simulink model "compressor"  (Simulink 7.4)
settings: Solver=ode45  StartTime=0.0  StopTime=85  RelTol=1e-3
values from neighbouring files (symbols this model uses):
  P_D = 0.9925    [MpcSetup.m]    (also in closedloop_setup.m = 1.12; test_linearization.m = P_D_init + delta_x(end,i))
  Ts = 0.05    [const_sim.m]    (also in test_linearization.m)
  u_out = uoff1(3)    [MpcSetup.m]    (also in closedloop_setup.m)
  x_init_lin = [0.916; 1.145; 0.152; 440; 0]    [closedloop_setup.m]    (also in test_linearization.m = [0.912; 1.17; 0.14; 465; 0])
libraries: dspsrcs4 x3
settings Model: Creator=chkajon  LastModifiedBy=chkajon

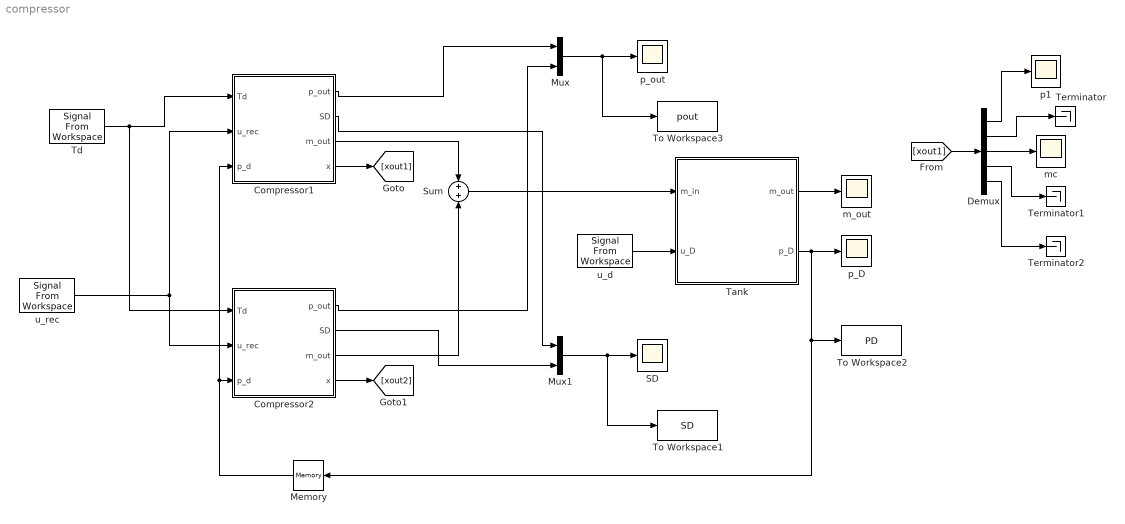
== system compressor ==
  Compressor1 : Subsystem  mask(Compressor){Td_off=0.304, u_in=0.405, u_out=u_out, u_rec=0, t_delay=1}
      mask prompts: Td_off "Torque offset"; u_in "Input valve setting"; u_out "Output valve setting"; u_rec "Recycle valve offset"; t_delay "Time delay"
      mask help: Compressor with tunable inputs.
  Compressor2 : Subsystem  mask(Compressor){Td_off=0.304, u_in=0.405, u_out=u_out, u_rec=0, t_delay=1}
      mask prompts: Td_off "Torque offset"; u_in "Input valve setting"; u_out "Output valve setting"; u_rec "Recycle valve offset"; t_delay "Time delay"
      mask help: Compressor with tunable inputs.
  Demux : Demux  Outputs=5
  Memory : Memory  X0=P_D  LinearizeMemory=on
  Mux : Mux  Inputs=2
  Mux1 : Mux  Inputs=2
  SD : Scope
      settings: YMin=-2.5  YMax=0
  Sum : Sum  OutDataType=fixdt(1, 16)  OutScaling=2^0
  Tank : Subsystem
  Td : dspsrcs4/Signal From Workspace  SystemSampleTime=-1  X=Td  Ts=Ts  nsamps=1  OutputAfterFinalValue=Holding final value  ignoreOrWarnInputAndFrameLengths=off
  Terminator : Terminator
  Terminator1 : Terminator
  Terminator2 : Terminator
  To Workspace1 : ToWorkspace  VariableName=SD  SampleTime=-1  SaveFormat=Structure With Time
  To Workspace2 : ToWorkspace  VariableName=PD  SampleTime=-1  SaveFormat=Structure With Time
  To Workspace3 : ToWorkspace  VariableName=pout  SampleTime=-1  SaveFormat=Structure With Time
  m_out : Scope
      settings: SaveName=ScopeData2
  mc : Scope
      settings: SaveName=ScopeData5
  p1 : Scope
      settings: SaveName=ScopeData4
  p_D : Scope
      settings: YMin=1.01  YMax=1.075  SaveName=ScopeData3
  p_out : Scope
  u_d : dspsrcs4/Signal From Workspace  SystemSampleTime=-1  X=u_d  Ts=Ts  nsamps=1  OutputAfterFinalValue=Holding final value  ignoreOrWarnInputAndFrameLengths=off
  u_rec : dspsrcs4/Signal From Workspace  SystemSampleTime=-1  X=u_rec  Ts=Ts  nsamps=1  OutputAfterFinalValue=Holding final value  ignoreOrWarnInputAndFrameLengths=off
  wires:
  Tank/1(m_out) -> m_out/1
  Tank/2(p_D) -> p_D/1, To Workspace2/1, Memory/1
  Compressor1/1(p_out) -> Mux/1
  Compressor1/2(SD) -> Mux1/1
  Compressor2/1(p_out) -> Mux/2
  Td/1 -> Compressor1/1(Td), Compressor2/1(Td)
  u_rec/1 -> Compressor1/2(u_rec), Compressor2/2(u_rec)
  u_d/1 -> Tank/2(u_D)
  Sum/1 -> Tank/1(m_in)
  Mux1/1 -> SD/1, To Workspace1/1
  Mux/1 -> p_out/1, To Workspace3/1
  Memory/1 -> Compressor1/3(p_d), Compressor2/3(p_d)
  Compressor1/3(m_out) -> Sum/1
  Compressor2/2(SD) -> Mux1/2
  Compressor2/3(m_out) -> Sum/2
  [xout1] -> Demux/1
  Compressor1/4(x) -> [xout1]
  Compressor2/4(x) -> [xout2]
  Demux/1 -> p1/1
  Demux/3 -> mc/1
  Demux/2 -> Terminator/1
  Demux/4 -> Terminator1/1
  Demux/5 -> Terminator2/1

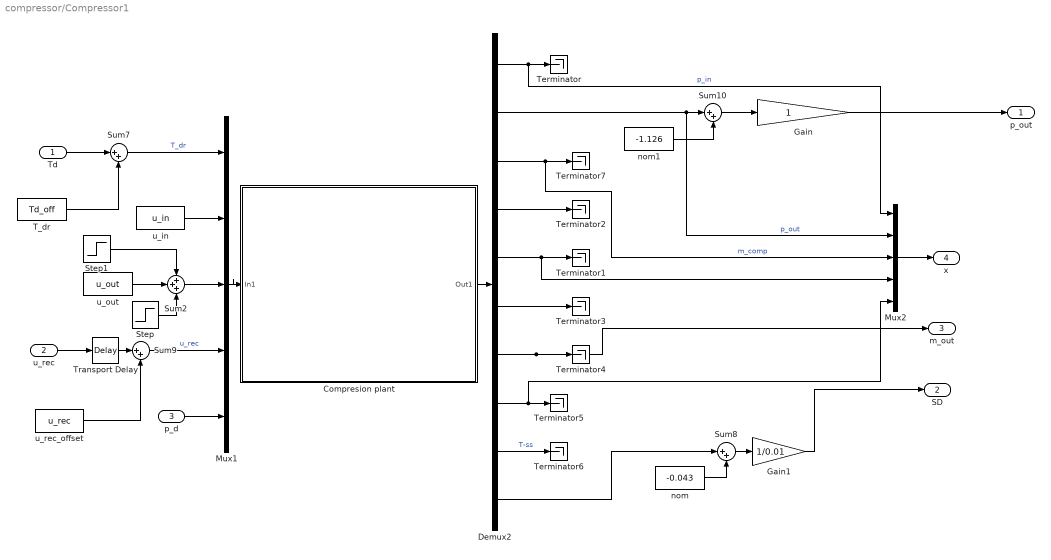
== system compressor/Compressor1 ==
  Td : Inport  OutDataType=fixdt(1, 16)  OutScaling=2^0
  u_rec : Inport  Port=2  OutDataType=fixdt(1, 16)  OutScaling=2^0
  p_d : Inport  Port=3  OutDataType=fixdt(1, 16)  OutScaling=2^0
  Compresion plant : Subsystem
      mask Display: image(imread('comp_plant.jpg'))
  Demux2 : Demux  Outputs=10
  Gain : Gain
  Gain1 : Gain  Gain=1/0.01
  Mux1 : Mux  Inputs=5
  Mux2 : Mux  Inputs=5
  Step : Step  Time=50  After=0  SampleTime=0
  Step1 : Step  Time=100  After=0  SampleTime=0
  Sum{7..10} (4 alike) : Sum  Inputs=|++
  Sum2 : Sum  Inputs=+++
  T_dr : Constant  Value=Td_off
  Terminator{,1..7} (8 alike) : Terminator
  Transport Delay : TransportDelay  DelayTime=t_delay
  nom : Constant  Value=-0.043
  nom1 : Constant  Value=-1.126
  u_in : Constant  Value=u_in
  u_out : Constant  Value=u_out
  u_rec_offset : Constant  Value=u_rec
  p_out : Outport  OutDataType=fixdt(1, 16)  OutScaling=2^0
  SD : Outport  Port=2  OutDataType=fixdt(1, 16)  OutScaling=2^0
  m_out : Outport  Port=3  OutDataType=fixdt(1, 16)  OutScaling=2^0
  x : Outport  Port=4  OutDataType=fixdt(1, 16)  OutScaling=2^0
  wires:
  Mux2/1 -> x/1
  Demux2/9 -> Terminator6/1  "T-ss"
  Sum2/1 -> Mux1/3
  Step/1 -> Sum2/3
  Transport Delay/1 -> Sum9/1
  p_d/1 -> Mux1/5
  Demux2/10 -> Sum8/1
  Gain1/1 -> SD/1
  Td/1 -> Sum7/1
  u_rec_offset/1 -> Sum9/2
  T_dr/1 -> Sum7/2
  Gain/1 -> p_out/1
  nom1/1 -> Sum10/2
  Sum10/1 -> Gain/1
  Demux2/5 -> Mux2/4, Terminator1/1
  Demux2/1 -> Mux2/1, Terminator/1  "p_in"
  Demux2/2 -> Mux2/2, Sum10/1  "p_out"
  Sum8/1 -> Gain1/1
  nom/1 -> Sum8/2
  Sum9/1 -> Mux1/4  "u_rec"
  Sum7/1 -> Mux1/1  "T_dr"
  u_rec/1 -> Transport Delay/1
  u_out/1 -> Sum2/2
  Demux2/7 -> Terminator4/1, m_out/1
  Demux2/8 -> Mux2/5, Terminator5/1
  Demux2/6 -> Terminator3/1
  u_in/1 -> Mux1/2
  Mux1/1 -> Compresion plant/1(In1)
  Compresion plant/1(Out1) -> Demux2/1
  Step1/1 -> Sum2/1
  Demux2/3 -> Mux2/3, Terminator7/1  "m_comp"
  Demux2/4 -> Terminator2/1

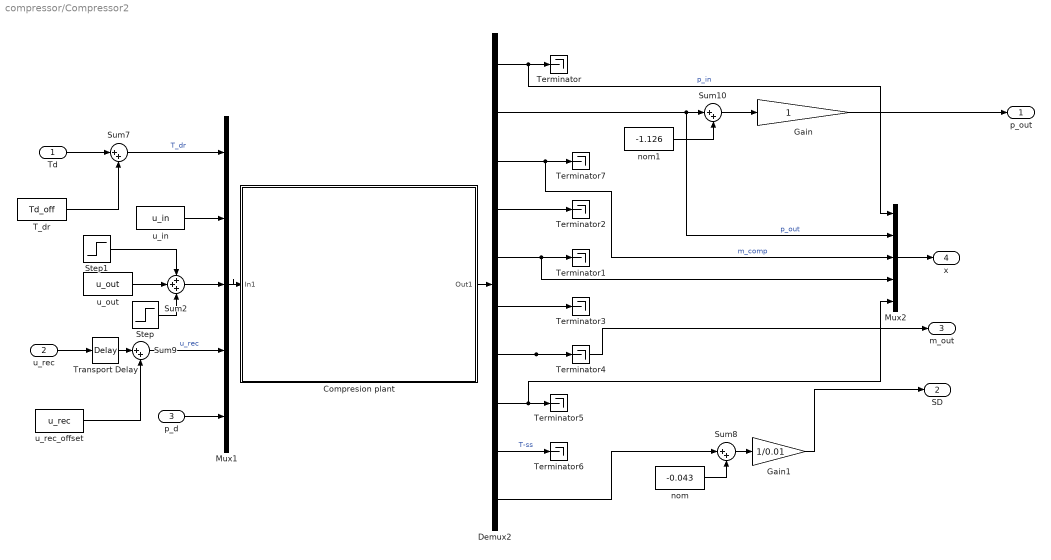
== system compressor/Compressor2 ==
  Td : Inport  OutDataType=fixdt(1, 16)  OutScaling=2^0
  u_rec : Inport  Port=2  OutDataType=fixdt(1, 16)  OutScaling=2^0
  p_d : Inport  Port=3  OutDataType=fixdt(1, 16)  OutScaling=2^0
  Compresion plant : Subsystem
      mask Display: image(imread('comp_plant.jpg'))
  Demux2 : Demux  Outputs=10
  Gain : Gain
  Gain1 : Gain  Gain=1/0.01
  Mux1 : Mux  Inputs=5
  Mux2 : Mux  Inputs=5
  Step : Step  Time=50  After=0  SampleTime=0
  Step1 : Step  Time=100  After=0  SampleTime=0
  Sum{7..10} (4 alike) : Sum  Inputs=|++
  Sum2 : Sum  Inputs=+++
  T_dr : Constant  Value=Td_off
  Terminator{,1..7} (8 alike) : Terminator
  Transport Delay : TransportDelay  DelayTime=t_delay
  nom : Constant  Value=-0.043
  nom1 : Constant  Value=-1.126
  u_in : Constant  Value=u_in
  u_out : Constant  Value=u_out
  u_rec_offset : Constant  Value=u_rec
  p_out : Outport  OutDataType=fixdt(1, 16)  OutScaling=2^0
  SD : Outport  Port=2  OutDataType=fixdt(1, 16)  OutScaling=2^0
  m_out : Outport  Port=3  OutDataType=fixdt(1, 16)  OutScaling=2^0
  x : Outport  Port=4  OutDataType=fixdt(1, 16)  OutScaling=2^0
  wires:
  Demux2/4 -> Terminator2/1
  Demux2/3 -> Terminator7/1, Mux2/3  "m_comp"
  Step1/1 -> Sum2/1
  Compresion plant/1(Out1) -> Demux2/1
  Mux1/1 -> Compresion plant/1(In1)
  u_in/1 -> Mux1/2
  Demux2/6 -> Terminator3/1
  Demux2/8 -> Terminator5/1, Mux2/5
  Demux2/7 -> m_out/1, Terminator4/1
  u_out/1 -> Sum2/2
  u_rec/1 -> Transport Delay/1
  Sum7/1 -> Mux1/1  "T_dr"
  Sum9/1 -> Mux1/4  "u_rec"
  nom/1 -> Sum8/2
  Sum8/1 -> Gain1/1
  Demux2/2 -> Sum10/1, Mux2/2  "p_out"
  Demux2/1 -> Terminator/1, Mux2/1  "p_in"
  Demux2/5 -> Terminator1/1, Mux2/4
  Sum10/1 -> Gain/1
  nom1/1 -> Sum10/2
  Gain/1 -> p_out/1
  T_dr/1 -> Sum7/2
  u_rec_offset/1 -> Sum9/2
  Td/1 -> Sum7/1
  Gain1/1 -> SD/1
  Demux2/10 -> Sum8/1
  p_d/1 -> Mux1/5
  Transport Delay/1 -> Sum9/1
  Step/1 -> Sum2/3
  Sum2/1 -> Mux1/3
  Demux2/9 -> Terminator6/1  "T-ss"
  Mux2/1 -> x/1

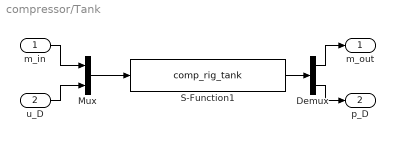
== system compressor/Tank ==
  m_in : Inport  OutDataType=fixdt(1, 16)  OutScaling=2^0
  u_D : Inport  Port=2  OutDataType=fixdt(1, 16)  OutScaling=2^0
  Demux : Demux  Outputs=2
  Mux : Mux  Inputs=2
  S-Function1 : S-Function  FunctionName=comp_rig_tank  Parameters=[], P_D  EnableBusSupport=off
  m_out : Outport  OutDataType=fixdt(1, 16)  OutScaling=2^0
  p_D : Outport  Port=2  OutDataType=fixdt(1, 16)  OutScaling=2^0
  wires:
  S-Function1/1 -> Demux/1
  Demux/1 -> m_out/1
  Demux/2 -> p_D/1
  Mux/1 -> S-Function1/1
  m_in/1 -> Mux/1
  u_D/1 -> Mux/2

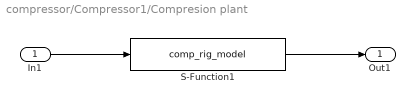
== system compressor/Compressor1/Compresion plant ==
  In1 : Inport
  S-Function1 : S-Function  FunctionName=comp_rig_model  Parameters=[], x_init_lin  EnableBusSupport=off
  Out1 : Outport
  wires:
  In1/1 -> S-Function1/1
  S-Function1/1 -> Out1/1

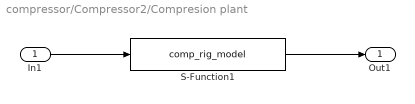
== system compressor/Compressor2/Compresion plant ==
  In1 : Inport
  S-Function1 : S-Function  FunctionName=comp_rig_model  Parameters=[], x_init_lin  EnableBusSupport=off
  Out1 : Outport
  wires:
  S-Function1/1 -> Out1/1
  In1/1 -> S-Function1/1
